simulink model "CIE237_4PAMS"  (R2025a)
settings: Solver=VariableStepAuto  StartTime=0.0  StopTime=1000  RelTol=1e-3
undefined symbols (not defined in the file): dspblkCoreblockFVToolHelper, gcbh
libraries: commsink2 x1, commrandsrc3 x1, dspsrcs4 x1, dspsigops x1
settings Model: Creator=compumarts  LastModifiedBy=compumarts

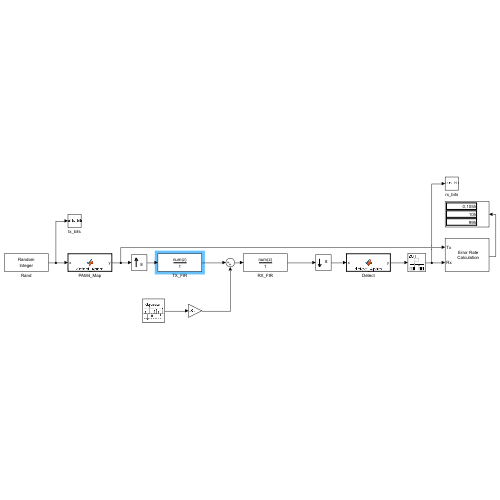
[thumbnail: Simulink's stored preview of the top-level diagram]
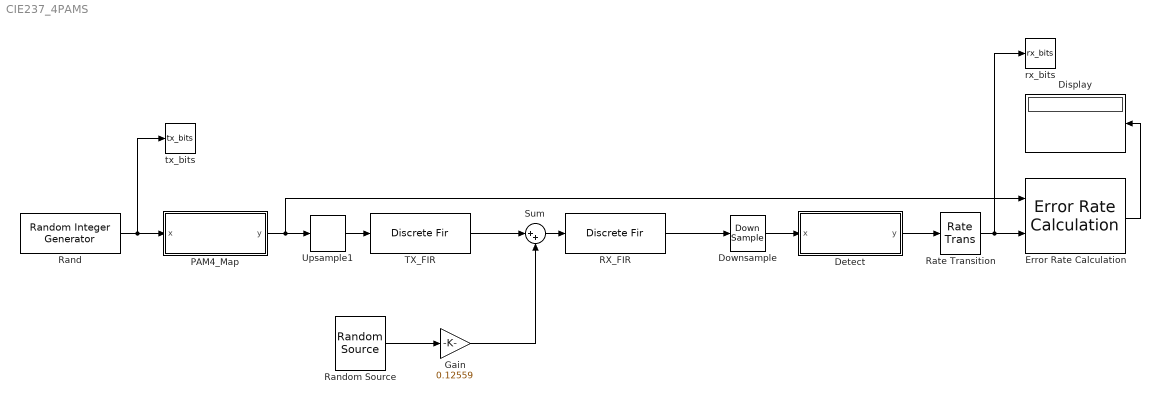
== system CIE237_4PAMS ==
  Detect : MATLAB Function  TreatAsAtomicUnit=on
  Display : Display
  Downsample : DownSample  N=8  AllowArbitraryFixedInput=on
  Error Rate Calculation : commsink2/Error Rate Calculation  N=6  st_delay=0  cp_mode=Entire frame  subframe=[]  PMode=Port  WsName=BER_out  RsMode2=off  stop=off  numErr=100  maxBits=1e6
  Gain : Gain  Gain=0.12559
  PAM4_Map : MATLAB Function  TreatAsAtomicUnit=on
  RX_FIR : DiscreteFir  LoadFcn=dspblkCoreblockFVToolHelper(gcbh,'load');  Coefficients=|  InputProcessing=Columns as channels (frame based)
      | [0.0011 -0.0027 -0.0058 -0.0070 -0.0053 -0.0008 0.0055 ...
      | 0.0116 0.0150 0.0134 0.0055 -0.0086 -0.0265 -0.0440 ...
      | -0.0555 -0.0549 -0.0375 -0.0005 0.0555 0.1263 0.2046 ...
      | 0.2808 0.3446 0.3870 0.4019 0.3870 0.3446 0.2808 ...
      | 0.2046 0.1263 0.0555 -0.0005 -0.0375 -0.0549 -0.0555 ...
      | -0.0440 -0.0265 -0.0086 0.0055 0.0134 0.0150 0.0116 ...
      | 0.0055 -0.0008 -0.0053 -0.0070 -0.0058 -0.0027 0.0011]
      settings: CopyFcn=dspblkCoreblockFVToolHelper(gcbh,'copy');  DeleteFcn=dspblkCoreblockFVToolHelper(gcbh,'close');  ModelCloseFcn=dspblkCoreblockFVToolHelper(gcbh,'close');  PreSaveFcn=dspblkCoreblockFVToolHelper(gcbh,'presave');  PostSaveFcn=dspblkCoreblockFVToolHelper(gcbh,'postsave');  CloseFcn=dspblkCoreblockFVToolHelper(gcbh,'close');
  Rand : commrandsrc3/Random Integer Generator  SetSize=4  SeedSource=Auto  Seed=0  SampleTime=1  SamplesPerFrame=1  OutputDataType=double  SimulateUsing=Interpreted execution
  Random Source : dspsrcs4/Random Source  SrcType=Gaussian  MinVal=0  MaxVal=1  MeanVal=0  VarVal=1  RepMode=Specify seed  rawSeed=1  IsInherit=off  SampTime=1  SampFrame=1  OutComplex=Real  DataType=double  SimulateUsing=Interpreted execution
  Rate Transition : RateTransition
  Sum : Sum  Inputs=|++
  TX_FIR : DiscreteFir  LoadFcn=dspblkCoreblockFVToolHelper(gcbh,'load');  Coefficients=|  InputProcessing=Columns as channels (frame based)
      | [0.0011 -0.0027 -0.0058 -0.0070 -0.0053 -0.0008 0.0055 ...
      | 0.0116 0.0150 0.0134 0.0055 -0.0086 -0.0265 -0.0440 ...
      | -0.0555 -0.0549 -0.0375 -0.0005 0.0555 0.1263 0.2046 ...
      | 0.2808 0.3446 0.3870 0.4019 0.3870 0.3446 0.2808 ...
      | 0.2046 0.1263 0.0555 -0.0005 -0.0375 -0.0549 -0.0555 ...
      | -0.0440 -0.0265 -0.0086 0.0055 0.0134 0.0150 0.0116 ...
      | 0.0055 -0.0008 -0.0053 -0.0070 -0.0058 -0.0027 0.0011]
      settings: CopyFcn=dspblkCoreblockFVToolHelper(gcbh,'copy');  DeleteFcn=dspblkCoreblockFVToolHelper(gcbh,'close');  ModelCloseFcn=dspblkCoreblockFVToolHelper(gcbh,'close');  PreSaveFcn=dspblkCoreblockFVToolHelper(gcbh,'presave');  PostSaveFcn=dspblkCoreblockFVToolHelper(gcbh,'postsave');  CloseFcn=dspblkCoreblockFVToolHelper(gcbh,'close');
  Upsample1 : dspsigops/Upsample  FactorSource=Dialog parameter  N=8  Nmax=16  phase=0  RateOptions=Allow multirate processing  ic=0  mode=Unused parameter value
  rx_bits : ToWorkspace  VariableName=rx_bits  SampleTime=-1
  tx_bits : ToWorkspace  VariableName=tx_bits  SampleTime=-1
  wires:
  Rand/1 -> tx_bits/1, PAM4_Map/1(x)
  PAM4_Map/1(y) -> Error Rate Calculation/1, Upsample1/1
  TX_FIR/1 -> Sum/1
  Sum/1 -> RX_FIR/1
  RX_FIR/1 -> Downsample/1
  Downsample/1 -> Detect/1(x)
  Upsample1/1 -> TX_FIR/1
  Random Source/1 -> Gain/1
  Gain/1 -> Sum/2
  Error Rate Calculation/1 -> Display/1
  Rate Transition/1 -> rx_bits/1, Error Rate Calculation/2
  Detect/1(y) -> Rate Transition/1

== matlab function CIE237_4PAMS/PAM4_Map ==
  data: x input; y output
function y = detect_4pam(x)
    thr1 = -0.14;
    thr2 = 0;
    thr3 = 0.14;
    
    y = zeros(size(x));
    
    y(x < thr1) = 0;
    y(x >= thr1 & x < thr2) = 1;
    y(x >= thr2 & x < thr3) = 2;
    y(x >= thr3) = 3;
end

== matlab function CIE237_4PAMS/Detect ==
  data: x input; y output
function y = detect_4pam(x)
if x < -2
    y = 0;

elseif x < 0
    y = 1;

elseif x < 2
    y = 2;

else
    y = 3;
end
